simulink model "MPPT_Using_Interleaved_Two_Inductor_Boost_Converter"  (R2019a)
settings: Solver=FixedStepAuto  StartTime=0.0  StopTime=.8  FixedStep=Tss  MaxStep=1e-6  RelTol=1e-3
undefined symbols (not defined in the file): Cin, Tpwm, Tss
libraries: powerlib x23, eePwmGenerator x2, re_lib x1, simulink x1
settings Model: SimulationMode=accelerator  Creator=asus  LastModifiedBy=asus
settings SolverCC: AlgebraicLoopSolver=LineSearch
settings DebuggingCC: UnconnectedInputMsg=none  UnconnectedOutputMsg=none  UnconnectedLineMsg=none

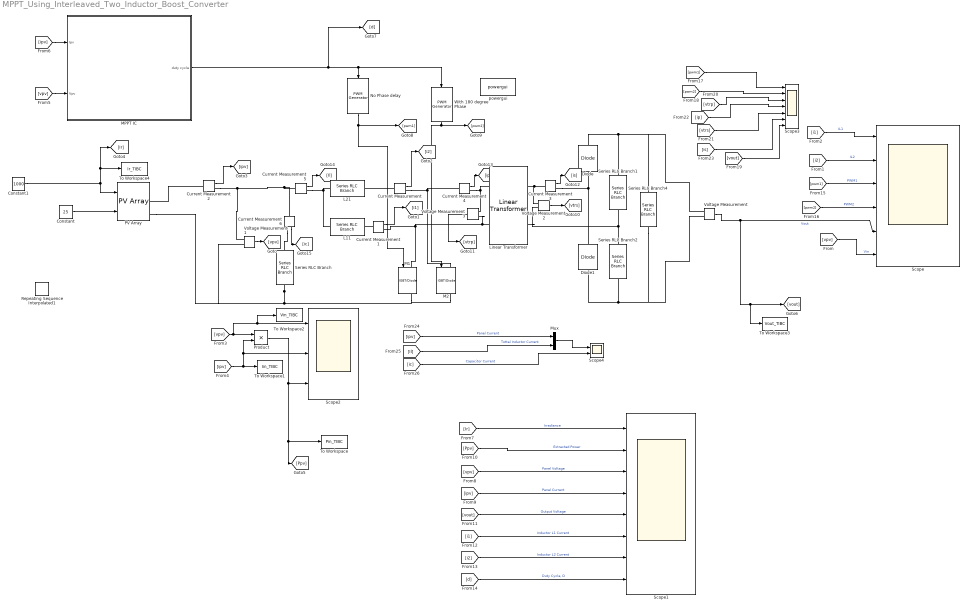
== system MPPT_Using_Interleaved_Two_Inductor_Boost_Converter ==
  Constant : Constant  Value=25
  Constant1 : Constant  Value=1000
  Current Measurement{,1..6} (7 alike) : powerlib/Measurements/Current Measurement  PhasorSimulation=off  OutputType=Complex  PSBequivalent=0
      settings: SourceProductName=Simscape Electrical
  Diode : powerlib/Power Electronics/Diode  Ron=1e-6  Lon=1e-9  Vf=0  IC=0  UseSnubber=0  Rs=500  Cs=250e-9  Measurements=off
      settings: SourceProductName=Simscape Electrical
  Diode1 : powerlib/Power Electronics/Diode  Ron=1e-6  Lon=1e-9  Vf=0  IC=0  UseSnubber=0  Rs=500  Cs=250e-9  Measurements=off
      settings: SourceProductName=Simscape Electrical
  L11 : powerlib/Elements/Series RLC Branch  LConnTagsString=__new0  RConnTagsString=__new0  BranchType=L  Resistance=1  Inductance=600e-6  SetiL0=off  InitialCurrent=0  Capacitance=Cin  Setx0=off  InitialVoltage=0  Measurements=None
      settings: SourceProductName=Simscape Electrical
  L21 : powerlib/Elements/Series RLC Branch  LConnTagsString=__new0  RConnTagsString=__new0  BranchType=L  Resistance=1  Inductance=600e-6  SetiL0=off  InitialCurrent=0  Capacitance=Cin  Setx0=off  InitialVoltage=0  Measurements=None
      settings: SourceProductName=Simscape Electrical
  Linear Transformer : powerlib/Elements/Linear Transformer  UNITS=SI  NominalPower=[ 500 1/Tpwm ]  winding1=[30 0 0]  winding2=[60 0 0]  ThreeWindings=off  winding3=[3.15e+05 0.7938 0.084225]  RmLm=[0 .5e-3]  Measurements=Winding voltages  DataType=on
      settings: SourceProductName=Simscape Electrical
  M1 : powerlib/Power Electronics/IGBT//Diode  Ron=1e-3  Rs=1e5  Cs=inf  Measurements=on
      settings: SourceProductName=Simscape Electrical
  M2 : powerlib/Power Electronics/IGBT//Diode  Ron=1e-3  Rs=1e5  Cs=inf  Measurements=on
      settings: SourceProductName=Simscape Electrical
  MPPT IC : Subsystem
  Mux : Mux  Inputs=2
  No Phase delay : eePwmGenerator/PWM Generator  CarrCount=Up  Tper=Tpwm  Ts=Tss
      settings: SourceProductName=Simscape Electrical
  PV Array : re_lib/Solar/PV Array  Npar=1  Nser=1  PlotType=array @ 25 deg.C & specified irradiances  S_vec="[ 1000 800 500  300 100 ]"  Temp_C_vec="[ 45 25  ]"  ModuleName=1Soltech 1STH-215-P  PlotWhenSelected=off  Pm=213.15  Ncell=60  Voc=36.3  Isc=7.84  Vm=29  Im=7.35  beta_Voc_pc=-0.36099  alpha_Isc_pc=0.102  beta_Voc=-0.13104  alpha_Isc=0.007997  IL=7.8649  I0=2.9259e-10  nI=0.98117  Rsh=313.3991  Rs=0.39383  BAL=on  Tc=1e-6  Tfilter=5e-5
      settings: SourceProductName=Simscape Electrical
  Product : Product
  Repeating Sequence Interpolated1 : simulink/Sources/Repeating Sequence Interpolated  OutValues=[800 800 1000 1000 500 500].'  TimeValues=[0 .8 .80001 1.6 1.60001 2.4].'  LookUpMeth=Interpolation-Use End Values  tsamp=0.01  OutMin=[]  OutMax=[]  OutDataTypeStr=double  OutputDataTypeScalingMode=double  OutDataType=fixdt(0,8)  OutScaling=2^-10
  Scope : Scope  NumInputPorts=6
  Scope1 : Scope  NumInputPorts=8
  Scope2 : Scope  NumInputPorts=3
  Scope3 : Scope  NumInputPorts=7
  Scope4 : Scope  NumInputPorts=2
  Series RLC Branch : powerlib/Elements/Series RLC Branch  LConnTagsString=__new0  RConnTagsString=__new0  BranchType=RC  Resistance=1e-3  Inductance=1e-3  SetiL0=off  InitialCurrent=0  Capacitance=100e-6  Setx0=off  InitialVoltage=0  Measurements=None
      settings: SourceProductName=Simscape Electrical
  Series RLC Branch1 : powerlib/Elements/Series RLC Branch  LConnTagsString=__new0  RConnTagsString=__new0  BranchType=C  Resistance=1  Inductance=1e-3  SetiL0=off  InitialCurrent=0  Capacitance=20e-06  Setx0=off  InitialVoltage=0  Measurements=Branch voltage
      settings: SourceProductName=Simscape Electrical
  Series RLC Branch2 : powerlib/Elements/Series RLC Branch  LConnTagsString=__new0  RConnTagsString=__new0  BranchType=C  Resistance=1  Inductance=1e-3  SetiL0=off  InitialCurrent=0  Capacitance=20e-6  Setx0=off  InitialVoltage=0  Measurements=Branch voltage
      settings: SourceProductName=Simscape Electrical
  Series RLC Branch4 : powerlib/Elements/Series RLC Branch  LConnTagsString=__new0  RConnTagsString=__new0  BranchType=R  Resistance=1000  Inductance=1e-3  SetiL0=off  InitialCurrent=0  Capacitance=470e-6  Setx0=off  InitialVoltage=0  Measurements=None
      settings: SourceProductName=Simscape Electrical
  To Workspace : ToWorkspace  VariableName=Pin_TIBC  SaveFormat=Timeseries  SampleTime=-1
  To Workspace1 : ToWorkspace  VariableName=Iin_TIBC  SaveFormat=Timeseries  SampleTime=-1
  To Workspace2 : ToWorkspace  VariableName=Vin_TIBC  SaveFormat=Timeseries  SampleTime=-1
  To Workspace3 : ToWorkspace  VariableName=Vout_TIBC  SaveFormat=Timeseries  SampleTime=-1
  To Workspace4 : ToWorkspace  VariableName=Ir_TIBC  SaveFormat=Timeseries  SampleTime=-1
  Voltage Measurement{,1..3} (4 alike) : powerlib/Measurements/Voltage Measurement  PhasorSimulation=off  OutputType=Complex  PSBequivalent=0
      settings: SourceProductName=Simscape Electrical
  With 180 degree Phase : eePwmGenerator/PWM Generator  CarrCount=Up  Tper=Tpwm  Ts=Tss
      link override Carrier counter: Tdelay=Tper*0.5
      settings: SourceProductName=Simscape Electrical
  powergui : powerlib/powergui  Priority=1  SimulationMode=Discrete  SampleTime=Tss  frequency=60  Iterations=50  frequencyindice=0  Pbase=100e6  ErrMax=1e-4  UnitsV=kV  UnitsW=MW  buscounter=0  FunctionMessages=off  echomessages=off  EnableUseOfTLC=off  CurrentSourceSwitches=off  DisableSnubberDevices=off  DisableRonSwitches=off  DisableVfSwitches=off  DisplayEquations=off  AutomaticDiscreteSolvers=off  SolverType=Tustin/Backward Euler (TBE)  Interpol=off  ExternalGateDelay=off  methode=off  Ts=100  x0status=blocks  SPID=on  SwTol=0  HookPort=off  NonlinearTolerance=0  nMaxIteration=15  ContinueOnMaxIteration=off  RestoreLinks=warning  ResistiveCurrentMeasurement=off  Frange=[0:2:500]  Ylog=off  Xlog=on  ShowGrid=off  save=off  variable=ZData  structure=0  ZoomFFT=off  StartTime=0.0  cycles=1  DisplayStyle=1  fundamental=60  FreqAxis=off  MaxFrequency=1000  frequencyindicesteady=1  RmsSteady=1  display=off
      settings: SourceProductName=Simscape Electrical
  wires:
  Voltage Measurement1/1 -> [vpv]
  Current Measurement1/1 -> [i1]
  Current Measurement/1 -> [i2]
  Constant/1 -> PV Array/2
  Current Measurement2/1 -> [ipv]
  [vpv] -> To Workspace2/1, Scope2/1, Product/1
  [ipv] -> To Workspace1/1, Scope2/2, Product/2
  Product/1 -> Scope2/3, To Workspace/1, [Ppv]
  With 180 degree Phase/1 -> [pwm2], M2/1
  [i1] -> Scope/1  "IL1"
  [pwm2] -> Scope/4  "PWM2"
  [pwm1] -> Scope/3  "PWM1"
  [i2] -> Scope/2  "IL2"
  [vpv] -> Scope/6  "Vin"
  Voltage Measurement/1 -> To Workspace3/1, [vout], Scope/5  "Vout"
  MPPT IC/1(duty cycle) -> No Phase delay/1, With 180 degree Phase/1, [d]
  [vpv] -> MPPT IC/2(Vpv)
  [ipv] -> MPPT IC/1(Ipv)
  [Ir] -> Scope1/1  "Irradiance"
  [vpv] -> Scope1/3  "Panel Voltage"
  [ipv] -> Scope1/4  "Panel Current"
  [Ppv] -> Scope1/2  "Extracted Power"
  [vout] -> Scope1/5  "Output Voltage"
  [i1] -> Scope1/6  "Inductor L1 Current"
  [i2] -> Scope1/7  "Inductor L2 Current"
  [d] -> Scope1/8  "Duty Cycle, D"
  No Phase delay/1 -> [pwm1], M1/1
  [pwm1] -> Scope3/1
  [pwm2] -> Scope3/2
  [vout] -> Scope3/7
  Voltage Measurement2/1 -> [vtrs]
  Voltage Measurement3/1 -> [vtrp]
  Current Measurement3/1 -> [is]
  Current Measurement4/1 -> [ip]
  [vtrp] -> Scope3/3
  [vtrs] -> Scope3/5
  [ip] -> Scope3/4
  [is] -> Scope3/6
  Constant1/1 -> To Workspace4/1, [Ir], PV Array/1
  Current Measurement5/1 -> [Il]
  Current Measurement6/1 -> [ic]
  [ic] -> Scope4/2  "Capacitor Current"
  [ipv] -> Mux/1  "Panel Current"
  [Il] -> Mux/2  "Tottal Inductor Current"
  Mux/1 -> Scope4/1
  connections:
  L21/LConn1 -- Current Measurement5/RConn1 -- L11/LConn1
  Series RLC Branch/RConn1 -- M2/RConn1 -- M1/RConn1 -- PV Array/RConn2 -- Voltage Measurement1/LConn2
  Current Measurement/RConn1 -- Current Measurement4/LConn1 -- M2/LConn1
  M1/LConn1 -- Current Measurement1/RConn1 -- Voltage Measurement3/LConn2 -- Linear Transformer/LConn2
  Diode1/RConn1 -- Current Measurement3/RConn1 -- Diode/LConn1
  Series RLC Branch2/LConn1 -- Voltage Measurement2/LConn2 -- Linear Transformer/RConn2 -- Series RLC Branch1/RConn1
  Diode/RConn1 -- Voltage Measurement/LConn1 -- Series RLC Branch4/LConn1 -- Series RLC Branch1/LConn1
  Current Measurement/LConn1 -- L21/RConn1
  Current Measurement1/LConn1 -- L11/RConn1
  Current Measurement2/LConn1 -- PV Array/RConn1
  Voltage Measurement/LConn2 -- Series RLC Branch4/RConn1 -- Diode1/LConn1 -- Series RLC Branch2/RConn1
  Linear Transformer/RConn1 -- Voltage Measurement2/LConn1 -- Current Measurement3/LConn1
  Linear Transformer/LConn1 -- Current Measurement4/RConn1 -- Voltage Measurement3/LConn1
  Current Measurement2/RConn1 -- Current Measurement6/LConn1 -- Current Measurement5/LConn1 -- Voltage Measurement1/LConn1
  Current Measurement6/RConn1 -- Series RLC Branch/LConn1

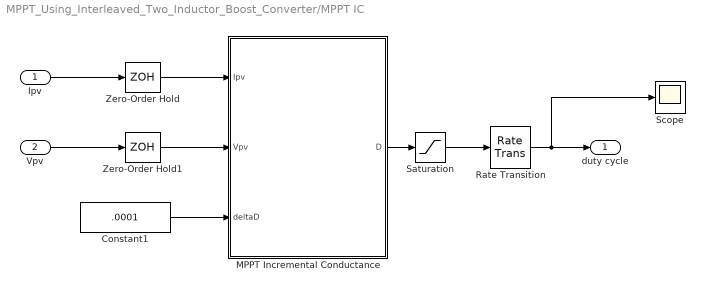
== system MPPT_Using_Interleaved_Two_Inductor_Boost_Converter/MPPT IC ==
  Ipv : Inport
  Vpv : Inport  Port=2
  Constant1 : Constant  Value=.0001
  MPPT Incremental Conductance : Stateflow chart  BlockKeywords=__PRM__SERIALIZED__DATA__:Stateflow Chart,Stateflow Diagram  TreatAsAtomicUnit=on
  Rate Transition : RateTransition
  Saturation : Saturate  UpperLimit=0.95  LowerLimit=.55
  Scope : Scope
  Zero-Order Hold : ZeroOrderHold  SampleTime=4*Tpwm
  Zero-Order Hold1 : ZeroOrderHold  SampleTime=4*Tpwm
  duty cycle : Outport
  wires:
  Constant1/1 -> MPPT Incremental Conductance/3(deltaD)
  Saturation/1 -> Rate Transition/1
  Rate Transition/1 -> Scope/1, duty cycle/1
  MPPT Incremental Conductance/1(D) -> Saturation/1
  Zero-Order Hold1/1 -> MPPT Incremental Conductance/2(Vpv)
  Zero-Order Hold/1 -> MPPT Incremental Conductance/1(Ipv)
  Ipv/1 -> Zero-Order Hold/1
  Vpv/1 -> Zero-Order Hold1/1

== stateflow chart MPPT_Using_Interleaved_Two_Inductor_Boost_Converter/MPPT IC/MPPT Incremental Conductance ==
  state SampleAndCalculate
    entry:
    dV=Vpv-Vpre;
    dI=Ipv-Ipre;
  state Init
    entry:
    Vpre=0;
    Ipre=0;
    D=0.9;
  state Decrease_Voltage
    entry:
    D=D+deltaD
  state Increase_Voltage
    entry:
    D=D-deltaD;
  state Increase_Voltage1
    entry:
    D=D-deltaD;
  state Decrease_Voltage1
    entry:
    D=D+deltaD;
  state RETURN
    entry:
    Vpre=Vpv;
    Ipre=Ipv;
  (junction 33) -> SampleAndCalculate
  (default) -> Init
  Init -> SampleAndCalculate
  SampleAndCalculate -> (junction 3) [order 1] : [dV~=0]
  SampleAndCalculate -> (junction 4) [order 2]
  (junction 3) -> (junction 24) [order 3]
  (junction 4) -> (junction 49) [order 3]
  (junction 4) -> Increase_Voltage1 [order 1] : [dI>0]
  (junction 3) -> Increase_Voltage [order 1] : [(Vpv*(dI/dV)+Ipv)>0]
  (junction 3) -> Decrease_Voltage [order 2] : [(Vpv*(dI/dV)+Ipv)<0]
  (junction 4) -> Decrease_Voltage1 [order 2] : [dI<0]
  RETURN -> (junction 33)
  (junction 49) -> RETURN
  (junction 24) -> RETURN
  Increase_Voltage -> RETURN
  Increase_Voltage1 -> RETURN
  Decrease_Voltage1 -> RETURN
  Decrease_Voltage -> RETURN
  data: Ipv input; Vpv input; deltaD input; Ipre local; dV local; dI local; Vpre local; D output
